simulink model "sampleModel1594"  (R2023a)
settings: Solver=VariableStepAuto  StartTime=0.0  StopTime=10.0  RelTol=1e-3
libraries: hdlsllib x1
settings Model: Creator=user1  LastModifiedBy=user1

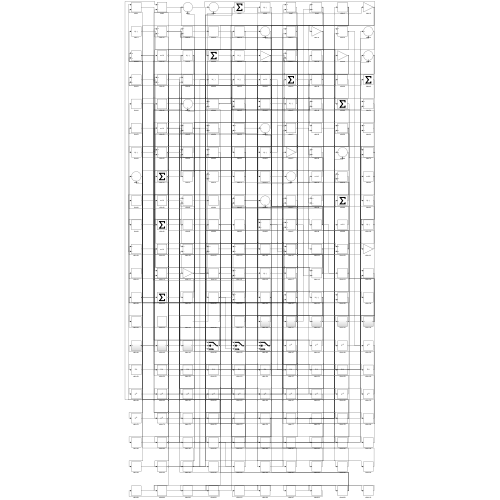
[thumbnail: Simulink's stored preview of the top-level diagram]
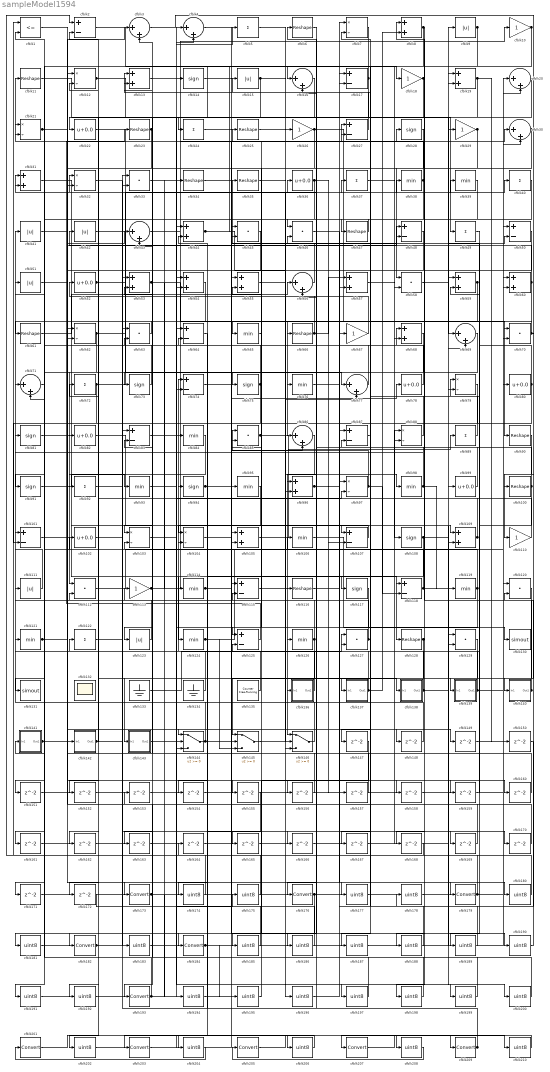
== system sampleModel1594 ==
  cfblk1 : RelationalOperator  Operator=<=  OutDataTypeStr=boolean  InputSameDT=off
  cfblk{10,18,26,29,67,110,113} (7 alike) : Gain
  cfblk{6,11,23,25,34..35,47,61,66,90,100,116,128} (13 alike) : Reshape
  cfblk{2,17,27,48,50,64,74,83,87,101,107,115,118,125} (14 alike) : Sum  Inputs=+-
  cfblk{22,36,52,78,80,82,99,102} (8 alike) : Bias  Bias=0.0  SaturateOnIntegerOverflow=off
  cfblk{7,12,21,32,62,79,88,97,103..104} (10 alike) : Product  Inputs=*/  RndMeth=Zero  SaturateOnIntegerOverflow=on
  cfblk{8,13,19,31,44,53..55,57,59..60,68,96,105,109} (15 alike) : Sum
  cfblk{38..39,65,76,84,93,95,98,106,114,119,121,124,126} (14 alike) : MinMax
  cfblk{14,28,73,75,81,91,94,108,117} (9 alike) : Signum
  cfblk{9,15,41..42,51,111,123} (7 alike) : Abs  SaturateOnIntegerOverflow=off
  cfblk{33,45..46,58,63,70,85,112,120,127,129} (11 alike) : DotProduct  OutDataTypeStr=Inherit: Inherit via internal rule
  cfblk{5,24,37,40,49,72,89,92,122} (9 alike) : Sum  Inputs=+
  cfblk130 : ToWorkspace  VariableName=simout  SaveFormat=Timeseries  SampleTime=-1
  cfblk131 : ToWorkspace  VariableName=simout  SaveFormat=Timeseries  SampleTime=-1
  cfblk132 : Scope
      settings: Floating=on
  cfblk133 : Ground
  cfblk134 : Ground
  cfblk135 : hdlsllib/Sources/Counter Free-Running  NumBits=16  tsamp=-1
  cfblk136 : Subsystem
      settings: LibrarySourceBlock=|
      | hdlsllib/Ports &
      | Subsystems/Subsystem
  cfblk137 : Subsystem
      settings: LibrarySourceBlock=|
      | hdlsllib/Ports &
      | Subsystems/Subsystem
  cfblk138 : Subsystem
      settings: LibrarySourceBlock=|
      | hdlsllib/Ports &
      | Subsystems/Subsystem
  cfblk139 : Subsystem
      settings: LibrarySourceBlock=|
      | hdlsllib/Ports &
      | Subsystems/Subsystem
  cfblk140 : Subsystem
      settings: LibrarySourceBlock=|
      | hdlsllib/Ports &
      | Subsystems/Subsystem
  cfblk141 : Subsystem
      settings: LibrarySourceBlock=|
      | hdlsllib/Ports &
      | Subsystems/Subsystem
  cfblk142 : Subsystem
      settings: LibrarySourceBlock=|
      | hdlsllib/Ports &
      | Subsystems/Subsystem
  cfblk143 : Subsystem
      settings: LibrarySourceBlock=|
      | hdlsllib/Ports &
      | Subsystems/Subsystem
  cfblk144 : Switch  SaturateOnIntegerOverflow=off  InputSameDT=off
  cfblk145 : Switch  SaturateOnIntegerOverflow=off  InputSameDT=off
  cfblk146 : Switch  SaturateOnIntegerOverflow=off  InputSameDT=off
  cfblk{147..172} (26 alike) : Delay  SampleTime=1
  cfblk{3..4,16,20,30,43,56,69,71,77,86} (11 alike) : Sum  Inputs=|++
  cfblk{173,176,179,182,184,193,201,203,205,207,209} (11 alike) : DataTypeConversion  SaturateOnIntegerOverflow=off  RndMeth=Floor
  cfblk{174..175,177..178,180..181,183,185..192,194..200,202,204,206,208,210} (27 alike) : DataTypeConversion  OutDataTypeStr=uint8  SaturateOnIntegerOverflow=off  RndMeth=Floor
  wires:
  cfblk129/1 -> cfblk176/1
  cfblk49/1 -> cfblk122/1
  cfblk88/1 -> cfblk15/1
  cfblk56/1 -> cfblk35/1
  cfblk75/1 -> cfblk112/1, cfblk53/2
  cfblk22/1 -> cfblk77/1
  cfblk44/1 -> cfblk18/1, cfblk116/1
  cfblk28/1 -> cfblk58/1
  cfblk85/1 -> cfblk89/1, cfblk118/1
  cfblk127/1 -> cfblk3/2, cfblk167/1
  cfblk125/1 -> cfblk23/1
  cfblk72/1 -> cfblk40/1, cfblk131/1
  cfblk16/1 -> cfblk103/1
  cfblk115/1 -> cfblk146/1
  cfblk109/1 -> cfblk68/1, cfblk12/2
  cfblk33/1 -> cfblk179/1
  cfblk23/1 -> cfblk43/2, cfblk152/1
  cfblk113/1 -> cfblk10/1, cfblk5/1
  cfblk62/1 -> cfblk38/1, cfblk82/1
  cfblk90/1 -> cfblk110/1
  cfblk99/1 -> cfblk31/1
  cfblk135/1 -> cfblk74/1
  cfblk13/1 -> cfblk14/1
  cfblk38/1 -> cfblk11/1, cfblk92/1
  cfblk12/1 -> cfblk49/1, cfblk44/1
  cfblk60/1 -> cfblk90/1, cfblk42/1
  cfblk66/1 -> cfblk25/1, cfblk57/1
  cfblk69/1 -> cfblk73/1
  cfblk26/1 -> cfblk70/1, cfblk192/1
  cfblk48/1 -> cfblk123/1
  cfblk112/1 -> cfblk19/1
  cfblk3/1 -> cfblk140/1(In1)
  cfblk104/1 -> cfblk78/1
  cfblk97/1 -> cfblk85/1, cfblk118/2
  cfblk86/1 -> cfblk126/1
  cfblk40/1 -> cfblk47/1
  cfblk108/1 -> cfblk154/1, cfblk200/1
  cfblk124/1 -> cfblk20/1, cfblk104/2, cfblk145/3
  cfblk138/1(Out1) -> cfblk59/1, cfblk21/2
  cfblk42/1 -> cfblk39/1
  cfblk107/1 -> cfblk104/1
  cfblk27/1 -> cfblk13/1
  cfblk58/1 -> cfblk29/1
  cfblk31/1 -> cfblk124/1
  cfblk64/1 -> cfblk184/1
  cfblk17/1 -> cfblk16/1, cfblk172/1
  cfblk59/1 -> cfblk86/1, cfblk163/1
  cfblk82/1 -> cfblk109/1
  cfblk98/1 -> cfblk6/1, cfblk119/1, cfblk81/1, cfblk63/2
  cfblk146/1 -> cfblk41/1
  cfblk111/1 -> cfblk71/1
  cfblk101/1 -> cfblk128/1
  cfblk81/1 -> cfblk107/1
  cfblk52/1 -> cfblk74/2, cfblk155/1
  cfblk15/1 -> cfblk98/1, cfblk144/3
  cfblk57/1 -> cfblk88/2
  cfblk139/1(Out1) -> cfblk80/1, cfblk112/2
  cfblk24/1 -> cfblk105/2
  cfblk68/1 -> cfblk91/1
  cfblk118/1 -> cfblk71/2, cfblk27/2, cfblk50/2
  cfblk70/1 -> cfblk100/1, cfblk65/1
  cfblk83/1 -> cfblk36/1
  cfblk134/1 -> cfblk31/2
  cfblk8/1 -> cfblk76/1, cfblk168/1
  cfblk136/1(Out1) -> cfblk101/1
  cfblk123/1 -> cfblk51/1
  cfblk128/1 -> cfblk145/1, cfblk143/1(In1)
  cfblk80/1 -> cfblk101/2, cfblk46/2
  cfblk84/1 -> cfblk182/1
  cfblk106/1 -> cfblk130/1
  cfblk105/1 -> cfblk17/2
  cfblk67/1 -> cfblk52/1
  cfblk126/1 -> cfblk113/1, cfblk162/1
  cfblk133/1 -> cfblk127/1
  cfblk19/1 -> cfblk22/1, cfblk150/1
  cfblk65/1 -> cfblk125/1
  cfblk110/1 -> cfblk7/2
  cfblk43/1 -> cfblk30/1
  cfblk140/1(Out1) -> cfblk79/1, cfblk8/1, cfblk139/1(In1)
  cfblk61/1 -> cfblk56/1
  cfblk122/1 -> cfblk144/1
  cfblk45/1 -> cfblk193/1
  cfblk37/1 -> cfblk68/2
  cfblk89/1 -> cfblk27/1
  cfblk137/1(Out1) -> cfblk121/1, cfblk83/2, cfblk8/2
  cfblk2/1 -> cfblk26/1
  cfblk121/1 -> cfblk3/1, cfblk43/1
  cfblk30/1 -> cfblk75/1, cfblk54/2
  cfblk1/1 -> cfblk173/1
  cfblk142/1(Out1) -> cfblk83/1, cfblk102/1
  cfblk14/1 -> cfblk115/1
  cfblk53/1 -> cfblk108/1, cfblk114/1
  cfblk35/1 -> cfblk146/2
  cfblk103/1 -> cfblk97/2
  cfblk96/1 -> cfblk157/1, cfblk158/1
  cfblk50/1 -> cfblk62/2
  cfblk5/1 -> cfblk77/2
  cfblk10/1 -> cfblk117/1, cfblk161/1
  cfblk6/1 -> cfblk96/1
  cfblk36/1 -> cfblk107/2, cfblk202/1
  cfblk18/1 -> cfblk96/2, cfblk188/1
  cfblk100/1 -> cfblk56/2, cfblk189/1
  cfblk78/1 -> cfblk32/1
  cfblk9/1 -> cfblk137/1(In1), cfblk58/2, cfblk146/3
  cfblk91/1 -> cfblk93/1
  cfblk7/1 -> cfblk24/1
  cfblk11/1 -> cfblk69/1
  cfblk117/1 -> cfblk144/2
  cfblk94/1 -> cfblk138/1(In1), cfblk109/2
  cfblk34/1 -> cfblk86/2
  cfblk119/1 -> cfblk94/1, cfblk136/1(In1)
  cfblk29/1 -> cfblk66/1, cfblk32/2
  cfblk77/1 -> cfblk21/1
  cfblk114/1 -> cfblk28/1, cfblk44/2
  cfblk73/1 -> cfblk2/2
  cfblk145/1 -> cfblk37/1
  cfblk63/1 -> cfblk61/1
  cfblk144/1 -> cfblk48/1, cfblk13/2, cfblk72/1
  cfblk141/1(Out1) -> cfblk142/1(In1), cfblk48/2
  cfblk21/1 -> cfblk145/2, cfblk148/1
  cfblk47/1 -> cfblk46/1
  cfblk120/1 -> cfblk147/1
  cfblk148/1 -> cfblk115/2
  cfblk93/1 -> cfblk149/1
  cfblk149/1 -> cfblk60/2
  cfblk71/1 -> cfblk151/1
  cfblk151/1 -> cfblk20/2
  cfblk152/1 -> cfblk97/1
  cfblk154/1 -> cfblk70/2
  cfblk74/1 -> cfblk156/1
  cfblk156/1 -> cfblk85/2
  cfblk157/1 -> cfblk62/1
  cfblk158/1 -> cfblk50/1
  cfblk51/1 -> cfblk159/1
  cfblk159/1 -> cfblk59/2
  cfblk46/1 -> cfblk160/1
  cfblk160/1 -> cfblk103/2
  cfblk161/1 -> cfblk69/2
  cfblk162/1 -> cfblk53/1
  cfblk163/1 -> cfblk57/2
  cfblk164/1 -> cfblk105/1
  cfblk32/1 -> cfblk165/1
  cfblk165/1 -> cfblk125/2
  cfblk102/1 -> cfblk166/1
  cfblk166/1 -> cfblk17/1
  cfblk167/1 -> cfblk88/1
  cfblk168/1 -> cfblk2/1
  cfblk76/1 -> cfblk169/1
  cfblk169/1 -> cfblk16/2
  cfblk143/1(Out1) -> cfblk170/1
  cfblk170/1 -> cfblk12/1
  cfblk54/1 -> cfblk171/1
  cfblk171/1 -> cfblk30/2
  cfblk173/1 -> cfblk99/1, cfblk194/1
  cfblk155/1 -> cfblk174/1
  cfblk174/1 -> cfblk1/1
  cfblk172/1 -> cfblk175/1
  cfblk175/1 -> cfblk1/2
  cfblk176/1 -> cfblk19/2, cfblk191/1
  cfblk41/1 -> cfblk177/1
  cfblk177/1 -> cfblk129/1
  cfblk150/1 -> cfblk178/1
  cfblk178/1 -> cfblk129/2
  cfblk179/1 -> cfblk127/2, cfblk141/1(In1)
  cfblk116/1 -> cfblk180/1
  cfblk180/1 -> cfblk33/1
  cfblk39/1 -> cfblk181/1
  cfblk181/1 -> cfblk33/2
  cfblk182/1 -> cfblk54/1, cfblk9/1
  cfblk92/1 -> cfblk183/1
  cfblk183/1 -> cfblk84/1
  cfblk184/1 -> cfblk79/2, cfblk60/1, cfblk195/1
  cfblk147/1 -> cfblk185/1
  cfblk185/1 -> cfblk64/1
  cfblk20/1 -> cfblk186/1
  cfblk186/1 -> cfblk64/2
  cfblk87/1 -> cfblk187/1
  cfblk187/1 -> cfblk120/1
  cfblk188/1 -> cfblk87/1
  cfblk189/1 -> cfblk87/2
  cfblk4/1 -> cfblk190/1
  cfblk190/1 -> cfblk120/2
  cfblk191/1 -> cfblk4/1
  cfblk192/1 -> cfblk4/2
  cfblk193/1 -> cfblk111/1, cfblk34/1
  cfblk194/1 -> cfblk45/1
  cfblk195/1 -> cfblk45/2
  cfblk55/1 -> cfblk196/1
  cfblk196/1 -> cfblk67/1
  cfblk25/1 -> cfblk197/1
  cfblk197/1 -> cfblk55/1
  cfblk79/1 -> cfblk198/1
  cfblk198/1 -> cfblk55/2
  cfblk153/1 -> cfblk199/1
  cfblk199/1 -> cfblk7/1
  cfblk200/1 -> cfblk153/1
  cfblk202/1 -> cfblk95/1
  cfblk95/1 -> cfblk204/1
  cfblk204/1 -> cfblk201/1
  cfblk201/1 -> cfblk206/1
  cfblk206/1 -> cfblk203/1
  cfblk207/1 -> cfblk209/1
  cfblk203/1 -> cfblk208/1
  cfblk208/1 -> cfblk205/1
  cfblk209/1 -> cfblk164/1, cfblk106/1, cfblk63/1
  cfblk205/1 -> cfblk210/1
  cfblk210/1 -> cfblk207/1

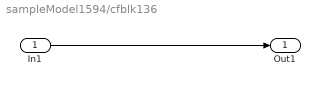
== system sampleModel1594/cfblk136 ==
  In1 : Inport
  Out1 : Outport
  wires:
  In1/1 -> Out1/1

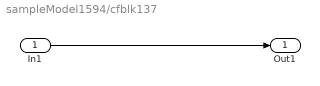
== system sampleModel1594/cfblk137 ==
  In1 : Inport
  Out1 : Outport
  wires:
  In1/1 -> Out1/1

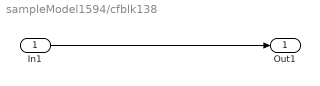
== system sampleModel1594/cfblk138 ==
  In1 : Inport
  Out1 : Outport
  wires:
  In1/1 -> Out1/1

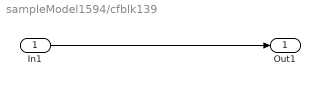
== system sampleModel1594/cfblk139 ==
  In1 : Inport
  Out1 : Outport
  wires:
  In1/1 -> Out1/1

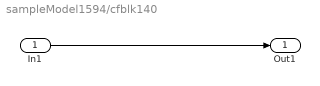
== system sampleModel1594/cfblk140 ==
  In1 : Inport
  Out1 : Outport
  wires:
  In1/1 -> Out1/1

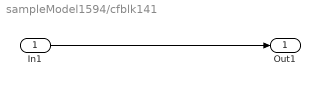
== system sampleModel1594/cfblk141 ==
  In1 : Inport
  Out1 : Outport
  wires:
  In1/1 -> Out1/1

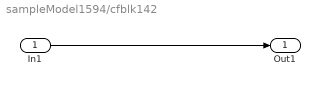
== system sampleModel1594/cfblk142 ==
  In1 : Inport
  Out1 : Outport
  wires:
  In1/1 -> Out1/1

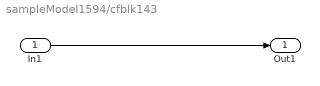
== system sampleModel1594/cfblk143 ==
  In1 : Inport
  Out1 : Outport
  wires:
  In1/1 -> Out1/1
